simulink model "line_follow"  (R2018b)
settings: Solver=ode3  StartTime=0.0  StopTime=10  RelTol=1e-3  EnableMultiTasking=on
libraries: legoev3lib x4
settings Model: FPTRunName=Active  ExtModeTrigDuration=2  Creator=wouter  LastModifiedBy=jloehnertz
settings SolverCC: PositivePriorityOrder=on
settings DataIOCC: LimitDataPoints=on  SaveFormat=Array
settings OptimizationCC: ExpressionDepthLimit=2147483647  LifeSpan=Inf  MaxStackSize=64
settings DebuggingCC: UnderspecifiedInitializationDetection=Classic  MergeDetectMultiDrivingBlocksExec=none  FcnCallInpInsideContextMsg=warning  AllowSymbolicDim=off  StateNameClashWarn=warning  SFUnexpectedBacktrackingDiag=warning  SFNoUnconditionalDefaultTransitionDiag=warning  SFExecutionAtInitializationDiag=none
settings HardwareCC: ProdBitPerPointer=32  ProdBitPerSizeT=32  ProdBitPerPtrDiffT=32  ProdLargestAtomicInteger=Long  ProdWordSize=32  ProdHWDeviceType=ARM Compatible->ARM 9  UseEmbeddedCoderFeatures=off  UseSimulinkCoderFeatures=off
settings ModelReferenceCC: PropagateSignalLabelsOutOfModel=off
settings SFSimCC: SimUseLocalCustomCode=off
settings RTWCC: SystemTargetFile=ert.tlc  HardwareBoard=LEGO MINDSTORMS EV3  TemplateMakefile=ert_default_tmf  GenerateReport=on  RTWVerbose=off  RTWUseLocalCustomCode=off  Toolchain=Sourcery G++ Lite v2009q3  BuildConfiguration=Faster Runs  LaunchReport=on
settings CodeAppCC: ForceParamTrailComments=on  OperatorAnnotations=on  StateflowObjectComments=on  MATLABSourceComments=on
settings ERTTargetCC: MultiwordLength=2048  ERTCustomFileBanners=off  SupportContinuousTime=on  SupportNonInlinedSFcns=on  RemoveResetFunc=off  SupportVariableSizeSignals=on  ModelStepFunctionPrototypeControlCompliant=off
settings ConfigComp: CovMetricSettings=dw  CovHtmlReporting=on  CovSaveCumulativeToWorkspaceVar=on  CovSaveSingleToWorkspaceVar=on  CovExternalEMLEnable=off  CovSFcnEnable=off

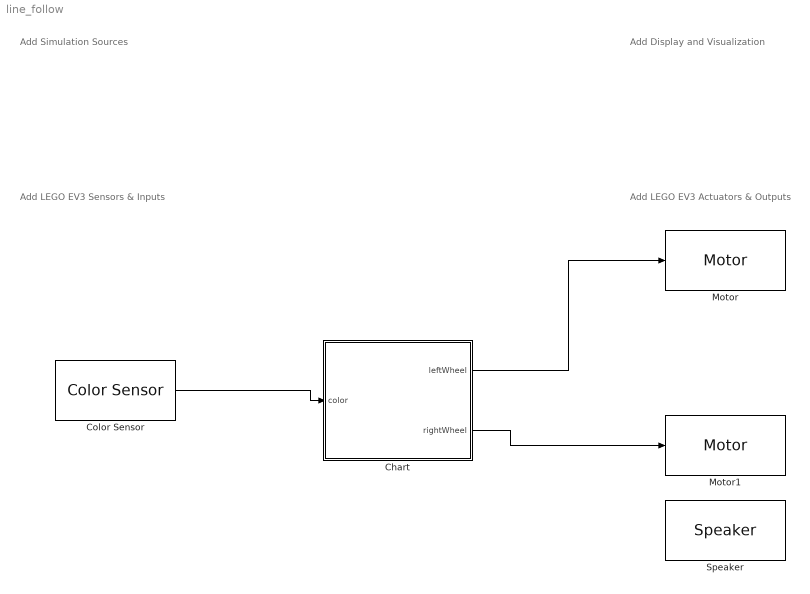
== system line_follow ==
  note: Add LEGO EV3 Sensors & Inputs
  note: Add LEGO EV3 Actuators & Outputs
  note: Add Display and Visualization
  note: Add Simulation Sources
  Chart : Stateflow chart  TreatAsAtomicUnit=on
  Color Sensor : legoev3lib/Color Sensor  portNumber=3  mode=Color  sampleTime=0.1
      settings: SourceProductName=Simulink Support Package for LEGO MINDSTORMS EV3 Hardware  SourceProductBaseCode=LEGOEV3
  Motor : legoev3lib/Motor  sportNumber=B  sstopAction=Brake
  Motor1 : legoev3lib/Motor  sportNumber=C  sstopAction=Brake
  Speaker : legoev3lib/Speaker  sinputMode=Frequency and volume  sspeakerFreq=100  sspeakerVolume=50  sspeakerDuration=500
      settings: SourceProductName=Simulink Support Package for LEGO MINDSTORMS EV3 Hardware  SourceProductBaseCode=LEGOEV3
  wires:
  Color Sensor/1 -> Chart/1(color)
  Chart/1(leftWheel) -> Motor/1
  Chart/2(rightWheel) -> Motor1/1

== stateflow chart line_follow/Chart ==
  state Flee2
    state Init
      entry:
      leftWheel = 0;
      rightWheel = 0;
    state Beep [commented out]
      entry:
      leftWheel = 0;
      lrightWheel = 0;
      speakerFreq = 600;
      speakerVol = 50;
    state Maneuver
      state TryLeft
        entry:
        lastDirection = 0;
        waitTime = waitTime * 2;
        state ALittleRight
          entry:
          leftWheel = scanSpeed;
          rightWheel = -scanSpeed / 2;
        state LeftCheck
          entry:
          leftWheel = -scanSpeed;
          rightWheel = scanSpeed / 2;
        state WaitForWhite
        (default) -> LeftCheck
        Flee2.Maneuver.TryLeft.WaitForWhite -> ALittleRight : [color ~= 1]
        LeftCheck -> Flee2.Maneuver.TryLeft.WaitForWhite [order 2] : [color == 1]
      state LastDirectionDecision
        entry: waitTime = 0.1;
      state Follow
        entry:
        leftWheel = driveSpeed;
        rightWheel = driveSpeed;
      state Stop
        entry:
        leftWheel = 0;
        rightWheel = 0;
      state TryRight
        entry:
        lastDirection = 1;
        waitTime = waitTime * 2;
        state RightCheck
          entry:
          leftWheel = scanSpeed;
          rightWheel = -scanSpeed / 2;
        state WaitForWhite
        state ALittleLeft
          entry:
          leftWheel = -scanSpeed;
          rightWheel = scanSpeed / 2;
        (default) -> RightCheck
        RightCheck -> Flee2.Maneuver.TryRight.WaitForWhite [order 2] : [color == 1]
        Flee2.Maneuver.TryRight.WaitForWhite -> ALittleLeft : [color ~= 1]
      (default) -> Follow
      LastDirectionDecision -> TryLeft [order 1] : [lastDirection == 0]
      Follow -> Stop : [color ~= 1]
      Stop -> LastDirectionDecision [order 1] : [color ~= 1]
      Stop -> Follow [order 2] : [color == 1]
      LastDirectionDecision -> TryRight [order 2] : [lastDirection == 1]
      ALittleRight -> Stop : [color == 1]
      ALittleLeft -> Stop : [color == 1]
      LeftCheck -> TryRight [order 1] : after(waitTime, sec)[color ~= 1]
      RightCheck -> TryLeft [order 1] : after(waitTime, sec)[color ~= 1]
    state RaiseFlag [commented out]
      entry:
      beep_volume = 0;
      raise_flag = 1;
    (default) -> Init
    Init -> Maneuver : [color == 1]
    Beep -> RaiseFlag [commented out] : after(0.5,sec)
  (default) -> Flee2
  data: color input; leftWheel output; rightWheel output; scanSpeed constant double =40; lastDirection local =0; waitTime local; driveSpeed constant double =40
